simulink model "lvxvjie_2_tf"  (R2023b)
settings: Solver=ode4  StartTime=0.0  StopTime=40  FixedStep=dt  RelTol=1e-3
undefined symbols (not defined in the file or in its folder): CPrt, CPrt_1, dt, EQ_intensity, EQ_sw, G_1, G_2, Gss, Gss_1, Klocate, Klocate1, KNrt_1, Koo, Kot, KPrt, KPrt_1, KRrt, locate, MPrt, MPrt_1, MRrt, T
libraries: simulink x1, sldrtlib x1
settings Model: Creator=icu327  LastModifiedBy=liangyu
settings DataIOCC: SaveFormat=Array  ReturnWorkspaceOutputs=off
settings DebuggingCC: UnconnectedInputMsg=warning  UnconnectedOutputMsg=warning  UnconnectedLineMsg=warning  ArithmeticOperatorsInVariantConditions=warning
settings HardwareCC: ProdBitPerLong=64  ProdHWDeviceType=Intel->x86-64 (Linux 64)
settings ModelReferenceCC: EnableRefExpFcnMdlSchedulingChecks=on
settings SFSimCC: CustomCodeUndefinedFunction=UseInterfaceOnly
settings RTWCC: Description=Simulink Desktop Real-Time  SystemTargetFile=sldrt.tlc  TemplateMakefile=sldrt.tmf  RTWCompilerOptimization=on
settings CodeAppCC: MaxIdLength=95  StateflowObjectComments=on
settings SimulinkDesktopRealTimeCC: TargetLibSuffix=_sldrt.a  TargetPreCompLibLocation=C:\Program Files\MATLAB\R2023b\toolbox\sldrt\lib\win64

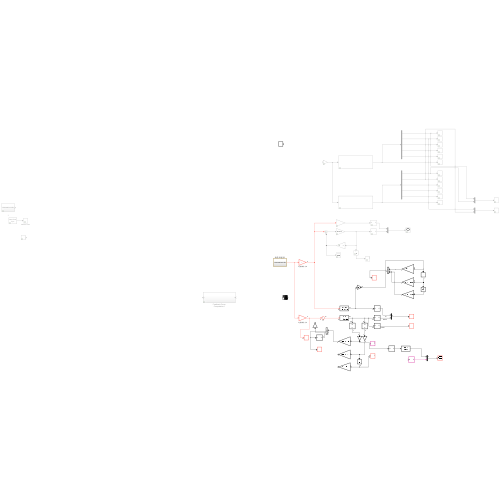
[thumbnail: Simulink's stored preview of the top-level diagram]
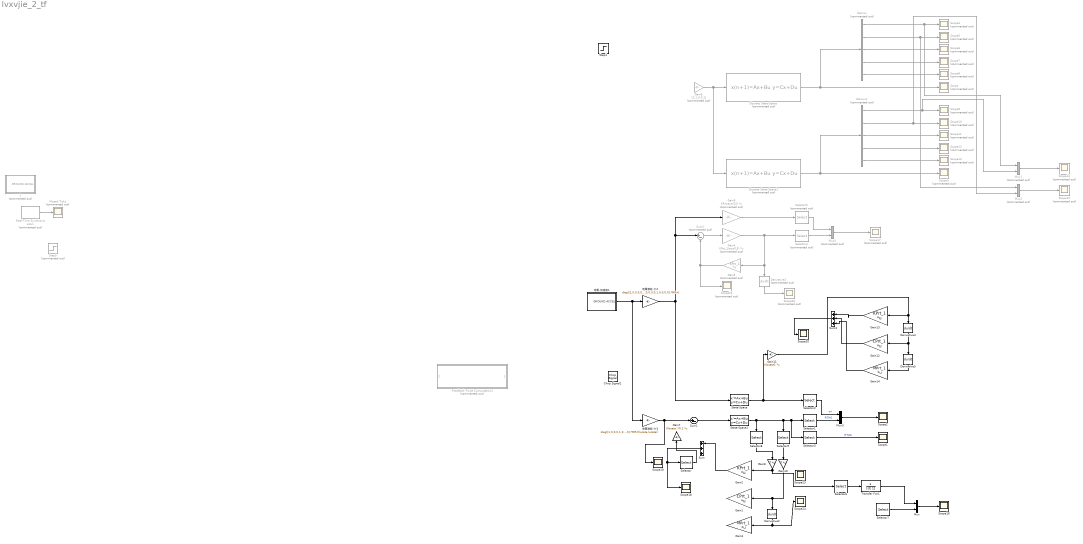
== system lvxvjie_2_tf ==
  " 1" : Subsystem  Commented=on
  " 地震-加速度1" : Subsystem
  Chirp Signal1 : simulink/Sources/Chirp Signal  f1=0.1  T=40  f2=10
  Demux : Demux  Commented=on  Outputs=5
  Demux1 : Demux  Commented=on  Outputs=5
  Derivative2 : Derivative
  Derivative3 : Derivative  Commented=on
  Derivative4 : Derivative
  Derivative5 : Derivative
  Discrete State-Space : DiscreteStateSpace  Commented=on  A=Gss.A  B=Gss.B  C=Gss.C  D=Gss.D  SampleTime=-1
  Discrete State-Space1 : DiscreteStateSpace  Commented=on  A=Gss_1.A  B=Gss_1.B  C=Gss_1.C  D=Gss_1.D  SampleTime=-1
  Feedback Force Computation1 : Subsystem  Commented=on
  Gain1 : Gain  Gain=CPrt_1  Multiplication=Matrix(K*u) (u vector)
  Gain10 : Gain  Gain=T  Multiplication=Matrix(K*u) (u vector)
  Gain11 : Gain  Gain=Klocate1  Multiplication=Matrix(K*u) (u vector)
  Gain12 : Gain  Gain=CPrt_1  Multiplication=Matrix(K*u) (u vector)
  Gain13 : Gain  Gain=KPrt_1  Multiplication=Matrix(K*u) (u vector)
  Gain14 : Gain  Gain=MPrt_1  Multiplication=Matrix(K*u) (u vector)
  Gain2 : Gain  Gain=KPrt_1  Multiplication=Matrix(K*u) (u vector)
  Gain3 : Gain  Gain=MPrt_1  Multiplication=Matrix(K*u) (u vector)
  Gain4 : Gain  Commented=on  Gain=KNrt_1\eye(15)  Multiplication=Matrix(K*u) (u vector)
  Gain5 : Gain  Commented=on  Gain=KPrt_1  Multiplication=Matrix(K*u) (u vector)
  Gain6 : Gain  Commented=on  Gain=[1,1,0,0,1]
  Gain7 : Gain  Gain=Klocate'.*0.2  Multiplication=Matrix(K*u) (u vector)
  Gain8 : Gain  Gain=T  Multiplication=Matrix(K*u) (u vector)
  Gain9 : Gain  Commented=on  Gain=KRrt\eye(15)  Multiplication=Matrix(K*u) (u vector)
  Missed Ticks : Scope  Commented=on
  Mux : Mux  Inputs=2
  Mux1 : Mux  Commented=on  Inputs=2
  Mux2 : Mux  Commented=on  Inputs=2
  Mux3 : Mux  Inputs=2
  Mux5 : Mux  Commented=on  Inputs=2
  Real-Time Synchronization : sldrtlib/Real-Time Synchronization  Commented=on  SampleTime=dt  MaxMissedTicks=10000  ShowMissedTicks=on  YieldWhenWaiting=off
  Scope{,3..15,17,22,26} (17 alike) : Scope  Commented=on
  Scope{1..2,16,18..20,23..24} (8 alike) : Scope
  Selector : Selector  InputPortWidth=6  IndexOptions=Index vector (dialog)  Indices=[1 2 3 4 5]  OutputSizes=1
  Selector1 : Selector  InputPortWidth=28  IndexOptions=Index vector (dialog)  Indices=[1]  OutputSizes=1
  Selector2 : Selector  InputPortWidth=15  IndexOptions=Index vector (dialog)  Indices=[1]  OutputSizes=1
  Selector3 : Selector  InputPortWidth=28  IndexOptions=Index vector (dialog)  Indices=[2]  OutputSizes=1
  Selector4 : Selector  Commented=on  InputPortWidth=15  IndexOptions=Index vector (dialog)  Indices=[1]  OutputSizes=1
  Selector5 : Selector  Commented=on  InputPortWidth=15  IndexOptions=Index vector (dialog)  Indices=[1]  OutputSizes=1
  Selector6 : Selector  InputPortWidth=6  IndexOptions=Index vector (dialog)  Indices=[1]  OutputSizes=1
  Selector7 : Selector  InputPortWidth=6  IndexOptions=Index vector (dialog)  Indices=[1]  OutputSizes=1
  Selector8 : Selector  InputPortWidth=28  IndexOptions=Index vector (dialog)  Indices=[1 2 5 6 7]  OutputSizes=1
  Selector9 : Selector  InputPortWidth=28  IndexOptions=Index vector (dialog)  Indices=[15 16 19 20 21]  OutputSizes=1
  State-Space : StateSpace  A=G_1.A  B=G_1.B  C=G_1.C  D=G_1.D  InitialCondition=0
  State-Space1 : StateSpace  A=G_2.A  B=G_2.B  C=G_2.C  D=G_2.D  InitialCondition=0
  Step1 : Step  SampleTime=0
  Step5 : Step  Commented=on  SampleTime=0
  Sum : Sum  Inputs=|+++
  Sum1 : Sum  Inputs=|+-
  Sum2 : Sum  Commented=on  Inputs=|+-
  Sum3 : Sum  Inputs=|+++
  Transfer Fcn1 : TransferFcn  Numerator=[1 0]  Denominator=[dt 1]
  地震激励-力2 : Gain  Gain=diag([1,0,0,0,0,1,0,0,0,0,1,0,0,0,0].*MRrt)
  地震激励-力3 : Gain  Gain=diag([1,0,0,0,1,0,0,0,0,1,0,0,0,0].*MRrt(locate,locate))
  wires:
  Real-Time Synchronization/1 -> Missed Ticks/1
  Discrete State-Space/1 -> Demux/1, Scope/1
  Demux/1 -> Mux1/1, Scope4/1
  Demux/2 -> Mux2/1, Scope5/1
  Demux/4 -> Scope7/1
  Demux/5 -> Scope8/1
  Demux1/5 -> Scope13/1
  Demux1/4 -> Scope12/1
  Demux1/1 -> Mux1/2, Scope9/1
  Discrete State-Space1/1 -> Demux1/1, Scope3/1
  Gain6/1 -> Discrete State-Space1/1, Discrete State-Space/1
  Demux1/3 -> Scope11/1
  Mux1/1 -> Scope14/1
  Mux2/1 -> Scope15/1
  Demux1/2 -> Mux2/2, Scope10/1
  Demux/3 -> Scope6/1
  " 地震-加速度1"/1(GROUND ACCEL) -> 地震激励-力3/1, 地震激励-力2/1
  Sum2/1 -> Gain4/1
  Gain5/1 -> Scope22/1, Sum2/2
  Gain9/1 -> Selector5/1
  Selector4/1 -> Mux5/2
  Selector5/1 -> Mux5/1
  Mux5/1 -> Scope17/1
  State-Space/1 -> Gain11/1, Selector2/1
  Sum1/1 -> State-Space1/1
  Mux3/1 -> Scope2/1
  Selector1/1 -> Mux3/2  "RTHS"
  地震激励-力2/1 -> State-Space/1, Sum2/1, Gain9/1
  Selector2/1 -> Mux3/1  "ori"
  Gain8/1 -> Selector6/1, Gain2/1
  Derivative2/1 -> Scope24/1, Gain3/1
  Gain4/1 -> Derivative3/1, Gain5/1, Selector4/1
  Derivative3/1 -> Scope26/1
  Sum/1 -> Scope18/1, Selector/1
  地震激励-力3/1 -> Scope19/1, Sum1/1
  Selector3/1 -> Scope1/1  "RTHS"
  State-Space1/1 -> Selector9/1, Selector3/1, Selector1/1, Selector8/1
  Selector/1 -> Gain7/1
  Selector6/1 -> Transfer Fcn1/1
  Selector7/1 -> Mux/2
  Mux/1 -> Scope16/1
  Transfer Fcn1/1 -> Mux/1
  Gain11/1 -> Derivative4/1, Gain13/1
  Gain12/1 -> Sum3/2
  Gain13/1 -> Sum3/1
  Gain14/1 -> Sum3/3
  Derivative5/1 -> Gain14/1
  Derivative4/1 -> Gain12/1, Derivative5/1
  Sum3/1 -> Scope20/1
  Selector8/1 -> Gain8/1
  Selector9/1 -> Gain10/1
  Gain10/1 -> Derivative2/1, Gain1/1
  Gain2/1 -> Sum/1

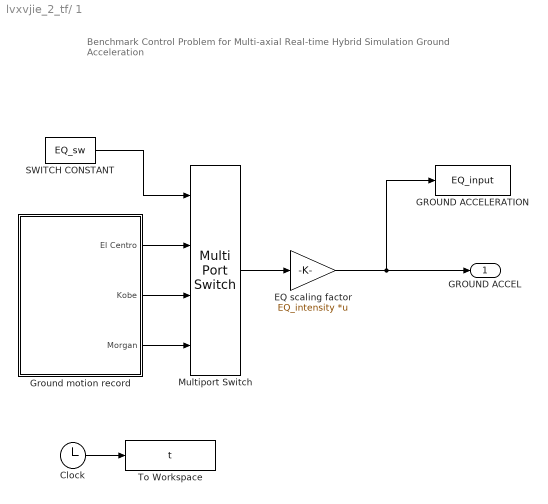
== system lvxvjie_2_tf/ 1 ==
  note: Benchmark Control Problem for
      | Multi-axial Real-time Hybrid Simulation
      | Ground Acceleration
  Clock : Clock
  EQ scaling factor : Gain  Gain=EQ_intensity  Multiplication=Matrix(K*u)
  GROUND ACCELERATION : ToWorkspace  VariableName=EQ_input  SampleTime=-1
      settings: Save2DSignal=2-D array (concatenate along first dimension)
  Ground motion record : Subsystem
  Multiport Switch : MultiPortSwitch  SaturateOnIntegerOverflow=off  InputSameDT=off
  SWITCH CONSTANT : Constant  Value=EQ_sw
  To Workspace : ToWorkspace  VariableName=t  SampleTime=dt
  GROUND ACCEL : Outport  VectorParamsAs1DForOutWhenUnconnected=off
  wires:
  Multiport Switch/1 -> EQ scaling factor/1
  EQ scaling factor/1 -> GROUND ACCELERATION/1, GROUND ACCEL/1
  Ground motion record/1(El Centro) -> Multiport Switch/2
  Ground motion record/2(Kobe) -> Multiport Switch/3
  Ground motion record/3(Morgan) -> Multiport Switch/4
  SWITCH CONSTANT/1 -> Multiport Switch/1
  Clock/1 -> To Workspace/1

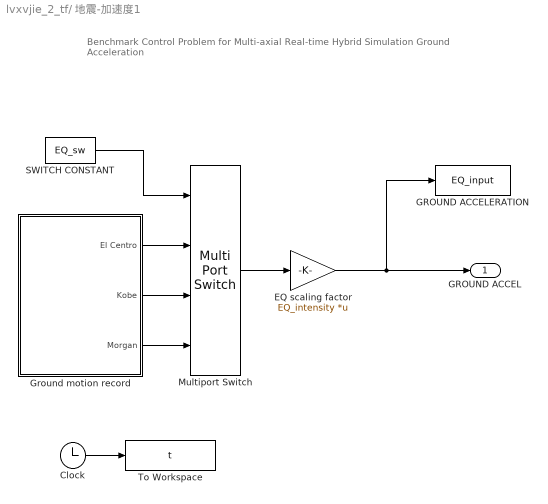
== system lvxvjie_2_tf/ 地震-加速度1 ==
  note: Benchmark Control Problem for
      | Multi-axial Real-time Hybrid Simulation
      | Ground Acceleration
  Clock : Clock
  EQ scaling factor : Gain  Gain=EQ_intensity  Multiplication=Matrix(K*u)
  GROUND ACCELERATION : ToWorkspace  VariableName=EQ_input  SampleTime=-1
      settings: Save2DSignal=2-D array (concatenate along first dimension)
  Ground motion record : Subsystem
  Multiport Switch : MultiPortSwitch  SaturateOnIntegerOverflow=off  InputSameDT=off
  SWITCH CONSTANT : Constant  Value=EQ_sw
  To Workspace : ToWorkspace  VariableName=t  SampleTime=dt
  GROUND ACCEL : Outport  VectorParamsAs1DForOutWhenUnconnected=off
  wires:
  Multiport Switch/1 -> EQ scaling factor/1
  EQ scaling factor/1 -> GROUND ACCELERATION/1, GROUND ACCEL/1
  Ground motion record/1(El Centro) -> Multiport Switch/2
  Ground motion record/2(Kobe) -> Multiport Switch/3
  Ground motion record/3(Morgan) -> Multiport Switch/4
  SWITCH CONSTANT/1 -> Multiport Switch/1
  Clock/1 -> To Workspace/1

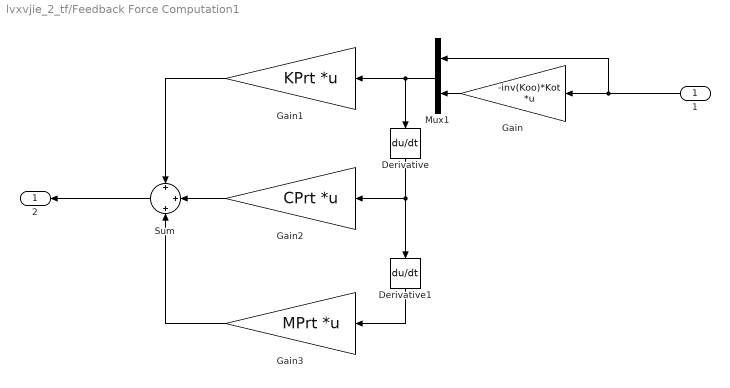
== system lvxvjie_2_tf/Feedback Force Computation1 ==
  1 : Inport
  Derivative : Derivative
  Derivative1 : Derivative
  Gain : Gain  Gain=-inv(Koo)*Kot  Multiplication=Matrix(K*u) (u vector)
  Gain1 : Gain  Gain=KPrt  Multiplication=Matrix(K*u) (u vector)
  Gain2 : Gain  Gain=CPrt  Multiplication=Matrix(K*u) (u vector)
  Gain3 : Gain  Gain=MPrt  Multiplication=Matrix(K*u) (u vector)
  Mux1 : Mux  Inputs=2
  Sum : Sum  Inputs=+|+|+
  2 : Outport  VectorParamsAs1DForOutWhenUnconnected=off
  wires:
  Gain/1 -> Mux1/2
  Derivative1/1 -> Gain3/1
  Gain2/1 -> Sum/2
  Derivative/1 -> Gain2/1, Derivative1/1
  Gain1/1 -> Sum/1
  1/1 -> Gain/1, Mux1/1
  Sum/1 -> 2/1
  Gain3/1 -> Sum/3
  Mux1/1 -> Derivative/1, Gain1/1

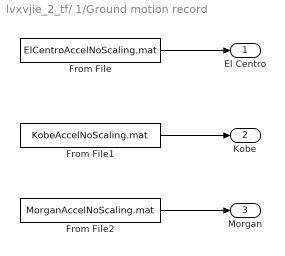
== system lvxvjie_2_tf/ 1/Ground motion record ==
  From File : FromFile  FileName=ElCentroAccelNoScaling.mat  SampleTime=dt
  From File1 : FromFile  FileName=KobeAccelNoScaling.mat  SampleTime=dt
  From File2 : FromFile  FileName=MorganAccelNoScaling.mat  SampleTime=dt
  El Centro : Outport
  Kobe : Outport  Port=2
  Morgan : Outport  Port=3
  wires:
  From File/1 -> El Centro/1
  From File2/1 -> Morgan/1
  From File1/1 -> Kobe/1

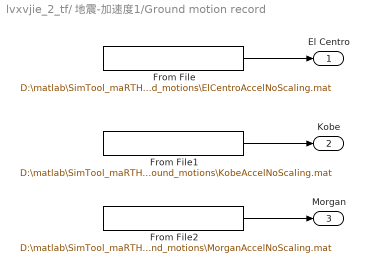
== system lvxvjie_2_tf/ 地震-加速度1/Ground motion record ==
  From File : FromFile  FileName=D:\matlab\SimTool_maRTHS_BenchM_V4 R2019b\Support_files\Ground_motions\ElCentroAccelNoScaling.mat  SampleTime=dt
  From File1 : FromFile  FileName=D:\matlab\SimTool_maRTHS_BenchM_V4 R2019b\Support_files\Ground_motions\KobeAccelNoScaling.mat  SampleTime=dt
  From File2 : FromFile  FileName=D:\matlab\SimTool_maRTHS_BenchM_V4 R2019b\Support_files\Ground_motions\MorganAccelNoScaling.mat  SampleTime=dt
  El Centro : Outport
  Kobe : Outport  Port=2
  Morgan : Outport  Port=3
  wires:
  From File/1 -> El Centro/1
  From File2/1 -> Morgan/1
  From File1/1 -> Kobe/1
